simulink model "VCMGCM1962020b_v2"  (R2020b)
settings: Solver=FixedStepDiscrete  StartTime=0.0  StopTime=10.0  FixedStep=0.005  RelTol=1e-3  EnableMultiTasking=on
PreLoadFcn:
  | try, model_open; catch, disp('Error occurred while executing model pre-load callback: model_open.m'); disp('Please assure that the MATLAB working directory is set to the model directory before opening.'); end
InitFcn:
  | try, model_open; catch, end
undefined symbols (not defined in the file): Bridge, GCM, H, raptor_get_param_eval, raptor_get_safe_string, raptor_xcp_function
libraries: Blocks_lib x1165, Raptor_lib x665, simulink x62, VCM_lib x5
(part 14 of 23)

== system VCMGCM1962020b_v2/Fgnd/Virtual Sensors/Charger/Off Board/OffBoardChgr ==
  Data : Inport
  Bus Selector : BusSelector  OutputSignals=Sensors.CAN.CCS.CCSM2IEV_Command.CCSChargerType.CCSChargerType [Enum]
  Header : Blocks_lib/Header  width=Portrait  addtext=''
  SMART_DC : simulink/Logic and Bit Operations/Compare To Constant  relop===  const=3  OutDataTypeStr=boolean
  Bool : Outport  VectorParamsAs1DForOutWhenUnconnected=off
  wires:
  Data/1 -> Bus Selector/1
  Bus Selector/1 -> SMART_DC/1  "<CCSChargerType [Enum]>"
  SMART_DC/1 -> Bool/1

== system VCMGCM1962020b_v2/Fgnd/Virtual Sensors/Charger/Off Board/OffBoardChgrIsoFault ==
  Data : Inport
  Bus Selector : BusSelector  OutputSignals=Sensors.CAN.CCS.CCSEVSE_DC_ChargeInfo1.CCSEVSEIsolationStatus.CCSEVSEIsolationStatusVld [Bool],Sensors.CAN.CCS.CCSEVSE_DC_ChargeInfo1.CCSEVSEIsolationStatus.CCSEVSEIsolationStatus [Enum]
  Fault : simulink/Logic and Bit Operations/Compare To Constant  relop===  const=2  OutDataTypeStr=boolean
  Header : Blocks_lib/Header  width=Portrait  addtext=''
  Zero-Order Hold : ZeroOrderHold  SampleTime=-1
  Vld : Outport  VectorParamsAs1DForOutWhenUnconnected=off
  Bool : Outport  Port=2  VectorParamsAs1DForOutWhenUnconnected=off
  wires:
  Fault/1 -> Bool/1
  Bus Selector/2 -> Fault/1  "<CCSEVSEIsolationStatus [Enum]>"
  Data/1 -> Bus Selector/1
  Zero-Order Hold/1 -> Vld/1
  Bus Selector/1 -> Zero-Order Hold/1  "<CCSEVSEIsolationStatusVld [Bool]>"

== system VCMGCM1962020b_v2/Fgnd/Virtual Sensors/Charger/Off Board/OffBoardChgrShutdown ==
  Data : Inport
  Bus Selector : BusSelector  OutputSignals=Sensors.CAN.CCS.CCSEVSE_DC_ChargeInfo1.CCSEVSEStatusCode.CCSEVSEStatusCode [Enum]
  EVSE Shutdown : simulink/Logic and Bit Operations/Compare To Constant  relop===  const=2  OutDataTypeStr=boolean
  Header : Blocks_lib/Header  width=Portrait  addtext=''
  Bool : Outport  VectorParamsAs1DForOutWhenUnconnected=off
  wires:
  EVSE Shutdown/1 -> Bool/1
  Data/1 -> Bus Selector/1
  Bus Selector/1 -> EVSE Shutdown/1  "<CCSEVSEStatusCode [Enum]>"

== system VCMGCM1962020b_v2/Fgnd/Virtual Sensors/Charger/On Board/OnBoardChgr ==
  note: TBC
  Data : Inport
  BASIC_AC : simulink/Logic and Bit Operations/Compare To Constant  relop===  const=1  OutDataTypeStr=boolean
  Bus Selector : BusSelector  Commented=on  OutputSignals=Sensors.CAN.CCS.CCSM2IEV_Command.CCSChargerType.CCSChargerType [Enum]
  Constant : Constant
  Header : Blocks_lib/Header  width=Portrait  addtext=''
  Bool : Outport  VectorParamsAs1DForOutWhenUnconnected=off
  wires:
  Data/1 -> Bus Selector/1
  BASIC_AC/1 -> Bool/1
  Constant/1 -> BASIC_AC/1

== system VCMGCM1962020b_v2/Fgnd/Virtual Sensors/Charger/On Board/OnBoardChgrFault ==
  Data : Inport
  Bus Selector1 : BusSelector  OutputSignals=Sensors.CAN.OnBoardChgr.ChgrCCSA.ChgrCCSAMsgVld [Bool],Sensors.CAN.OnBoardChgr.ChgrCCSA.ChgrChrgr_hardware_protect.ChgrChrgr_hardware_protect [enum],Sensors.CAN.OnBoardChgr.ChgrCCSA.ChgrChargr_temp_flag.ChgrChargr_temp_flag [enum],Sensors.CAN.OnBoardChgr.ChgrCCSA.ChgrChrgr_input_volt_flag.ChgrChrgr_input_volt_flag [enum],Sensors.CAN.OnBoardChgr.ChgrCCSA.ChgrChrgr_input_volt_flag.ChgrChrgr_input_volt_flag [enum],Sensors.CAN.OnBoardChgr.ChgrCCSA.ChgrChrgr_input_volt_flag.ChgrChrgr_input_volt_flag [enum]
  CntrSat : Blocks_lib/CntrSat  init=0  inc=1  typ=uint16  relop=>=  th_nam='OnBoardChgrFaultVldWaitTime'  th_gain=samptime  th_units='sec'  th_help='On-board charger fault valid wait time'  th_group='Virtual Sensors | Charger'
  Header : Blocks_lib/Header  width=Portrait  addtext=''
  Logical Operator1 : Logic  OutDataTypeStr=boolean
  Logical Operator2 : Logic  Operator=NOT  Inputs=1  OutDataTypeStr=boolean
  Logical Operator3 : Logic  Operator=OR  Inputs=5  OutDataTypeStr=boolean
  Vld : Outport  VectorParamsAs1DForOutWhenUnconnected=off
  Bool : Outport  Port=2  VectorParamsAs1DForOutWhenUnconnected=off
  wires:
  Data/1 -> Bus Selector1/1
  Bus Selector1/1 -> Vld/1, Logical Operator1/1  "<ChgrCCSAMsgVld [Bool]>"
  Logical Operator2/1 -> CntrSat/2
  Logical Operator1/1 -> Logical Operator2/1, CntrSat/1
  CntrSat/1 -> Bool/1
  Logical Operator3/1 -> Logical Operator1/2
  Bus Selector1/2 -> Logical Operator3/1  "<ChgrChrgr_hardware_protect [enum]>"
  Bus Selector1/3 -> Logical Operator3/2  "<ChgrChargr_temp_flag [enum]>"
  Bus Selector1/4 -> Logical Operator3/3  "<ChgrChrgr_input_volt_flag [enum]>"
  Bus Selector1/5 -> Logical Operator3/4  "<ChgrChrgr_input_volt_flag [enum]>"
  Bus Selector1/6 -> Logical Operator3/5  "<ChgrChrgr_input_volt_flag [enum]>"

== system VCMGCM1962020b_v2/Fgnd/Virtual Sensors/Driver Inputs/APP/Learn-Up Enable ==
  Data : Inport
  Bus Selector : BusSelector  OutputSignals=VirtualSensors.Spd.VehSpd [kph]
  Header : Blocks_lib/Header  width=Portrait  addtext=''
  Relational Operator : RelationalOperator  Operator=<=  OutDataTypeStr=boolean  RndMeth=Nearest
  raptor_adjustment : Raptor_lib/Data Storage/raptor_adjustment  paramName='APPLearnUpEnblVehSpdThr'  nameSource=Parameter  initValue=0  dataType=double  storage=Calibration  calDispType=Number  calEnum={}  calGain=1.0  calOffset=0.0  calMax=inf  calMin=-inf  calFormat='-1'  calUnit='kph'  calHelp='Learn-up strategy enable vehicle speed threshold'  calAccess=1  calFunction='Virtual Sensors | Driver Input'  calDispHeaders=off  calColHeaders={'Col1' 'Col2' 'Col3'}  calRowHeaders={'Row1' 'Row2' 'Row3'}
      settings: SourceProductName=Raptor
  Bool : Outport  VectorParamsAs1DForOutWhenUnconnected=off
  wires:
  Bus Selector/1 -> Relational Operator/1  "<VehSpd [kph]>"
  Data/1 -> Bus Selector/1
  Relational Operator/1 -> Bool/1
  raptor_adjustment/1 -> Relational Operator/2

== system VCMGCM1962020b_v2/Fgnd/Virtual Sensors/Driver Inputs/Brk/BrkPos ==
  Data : Inport
  Arb : Blocks_lib/Arb  nam='BrkPos'  units='%'  eqn='(u(1) + u(2)) / 2'  minmax=min  samptime=samptime
  Bus Selector : BusSelector  OutputSignals=Sensors.Sensors.Driver.BrkPos1.BrkPos1Vld [Bool],Sensors.Sensors.Driver.BrkPos2.BrkPos2Vld [Bool],Sensors.Sensors.Driver.BrkPos1.BrkPos1 [%],Sensors.Sensors.Driver.BrkPos2.BrkPos2 [%]
  Bus Selector2 : BusSelector  OutputSignals=Sensors.Sensors.Driver.APP1.APP1Vld [Bool],Sensors.Sensors.Driver.APP1ADC [ADC]
  Bus Selector3 : BusSelector  OutputSignals=Sensors.Sensors.Driver.APP2.APP2Vld [Bool],Sensors.Sensors.Driver.APP2ADC [ADC]
  Ddbnd(PctInpt) : Blocks_lib/Ddbnd(PctInpt)  nam='BrkPos'  group='Virtual Sensors | Driver Input'
  Header : Blocks_lib/Header  width=Portrait  addtext=''
  Learn-Up Enable : Subsystem
  Meas&Ovrd : Blocks_lib/Meas&Ovrd  nam='BrkPos'  name_source=Parameter  view_as=Number  enum_struct={}  gain=1  min=-inf  max=inf  precision=''  units='%'  help='Accelerator pedal position'  group='Virtual Sensors | Driver Input'
  SnsLinPctAdapt : Blocks_lib/SnsLinPctAdapt  nam='BrkPos1'  group='Virtual Sensors | Driver Input'  samptime=samptime
  SnsLinPctAdapt1 : Blocks_lib/SnsLinPctAdapt  nam='BrkPos2'  group='Virtual Sensors | Driver Input'  samptime=samptime
  Vld : Outport  VectorParamsAs1DForOutWhenUnconnected=off
  % : Outport  Port=2  VectorParamsAs1DForOutWhenUnconnected=off
  wires:
  Data/1 -> Bus Selector3/1, Learn-Up Enable/1(Data), Bus Selector2/1, Bus Selector/1
  Arb/1 -> Vld/1
  Meas&Ovrd/1 -> %/1
  Bus Selector3/2 -> SnsLinPctAdapt1/2  "<APP2ADC [ADC]>"
  Bus Selector3/1 -> SnsLinPctAdapt1/1  "<APP2Vld [Bool]>"
  Learn-Up Enable/1(Bool) -> SnsLinPctAdapt1/3, SnsLinPctAdapt/3
  Bus Selector2/2 -> SnsLinPctAdapt/2  "<APP1ADC [ADC]>"
  Bus Selector2/1 -> SnsLinPctAdapt/1  "<APP1Vld [Bool]>"
  Bus Selector/4 -> Arb/4  "<BrkPos2 [%]>"
  Bus Selector/3 -> Arb/3  "<BrkPos1 [%]>"
  Bus Selector/2 -> Arb/2  "<BrkPos2Vld [Bool]>"
  Bus Selector/1 -> Arb/1  "<BrkPos1Vld [Bool]>"
  Arb/2 -> Ddbnd(PctInpt)/1
  Ddbnd(PctInpt)/1 -> Meas&Ovrd/1

== system VCMGCM1962020b_v2/Fgnd/Virtual Sensors/PDU/HVBusVolt/HV Bus Voltage ==
  Data : Inport
  Avg : Subsystem
  Demux : Demux
  Diag : Subsystem
  Function-Call Generator : simulink/Ports & Subsystems/Function-Call Generator  sample_time=-1  numberOfIterations=1  DisallowWideOutput=off
  Header : Blocks_lib/Header  width=Portrait  addtext=''
  Reset : Subsystem
  "Sum, Max, Min" : Subsystem
  Vld : Outport  VectorParamsAs1DForOutWhenUnconnected=off
  V : Outport  Port=2  VectorParamsAs1DForOutWhenUnconnected=off
  wires:
  Function-Call Generator/1 -> Demux/1
  Demux/2 -> "Sum, Max, Min"/Trigger
  Demux/3 -> Avg/Trigger
  Demux/4 -> Diag/Trigger
  Demux/1 -> Reset/Trigger
  Avg/2(V) -> Diag/1(V), V/1
  Avg/1(Vld) -> Vld/1
  Data/1 -> "Sum, Max, Min"/1(Data)

== system VCMGCM1962020b_v2/Fgnd/Virtual Sensors/Vehicle/Range/CntrLoop ==
  Compare To Constant : simulink/Logic and Bit Operations/Compare To Constant  relop=>=  const=rstval  OutDataTypeStr=boolean
  Constant : Constant  Value=init  OutDataTypeStr=uint16
  Header : Blocks_lib/Header  width=Portrait  addtext=''
  Increment Real World : simulink/Additional Math & Discrete/Additional Math: Increment - Decrement/Increment Real World
      settings: SourceProductBaseCode=SL
  Multiport Switch : MultiPortSwitch  DataPortOrder=Zero-based contiguous  Inputs=2  zeroidx=on  InputSameDT=on
  Unit Delay : UnitDelay  InitialCondition=init  SampleTime=-1  HasFrameUpgradeWarning=on
  Count : Outport  VectorParamsAs1DForOutWhenUnconnected=off
  wires:
  Constant/1 -> Multiport Switch/3
  Increment Real World/1 -> Multiport Switch/2
  Compare To Constant/1 -> Multiport Switch/1
  Multiport Switch/1 -> Unit Delay/1, Count/1
  Unit Delay/1 -> Compare To Constant/1, Increment Real World/1

== system VCMGCM1962020b_v2/Fgnd/Virtual Sensors/Vehicle/Range/RangeGain ==
  Odom : Inport
  data : Inport  Port=2
  Rst : Inport  Port=3
  Init : Inport  Port=4
  Enable : EnablePort
  Add : Sum  Inputs=+-
  Add2 : Sum  Inputs=-+
  Bus Selector : BusSelector  OutputSignals=VirtualSensors.Batt.BattSOC [%]
  Bus Selector1 : BusSelector  OutputSignals=Control.Mode.StartStop.RunMode [Bool]
  CntrLoop : Subsystem  TreatAsAtomicUnit=on  mask(CntrLoop){init=0, typ=uint16, rstval=2000}
      mask prompts: init "Initial Value"; typ "Data Type"; rstval "Reset at:"
      mask init:
      | cb = gcb;
      | 
      | % --- Parameter Setting
      | set_param([cb '/Constant'], 'OutDataTypeStr', typ);
      mask TypeOptions typ: double | single | int8 | uint8 | int16 | uint16 | int32 | uint32 | boolean
      mask Display: disp(['Loop Counter\nReset at ' num2str(rstval)]);
  Compare To Constant : simulink/Logic and Bit Operations/Compare To Constant  relop=~=  const=0  OutDataTypeStr=boolean
  Header : Blocks_lib/Header  width=Portrait  addtext=''
  Moving Average : Subsystem
  Mux : Mux  Inputs=2
  Saturation : Saturate  UpperLimit=100  LowerLimit=0
  Subsystem : Subsystem
  Unit Delay : UnitDelay  SampleTime=-1  HasFrameUpgradeWarning=on
  Unit Delay1 : UnitDelay  SampleTime=-1  HasFrameUpgradeWarning=on
  raptor_measurement : Raptor_lib/Data Storage/raptor_measurement  paramName='RangeEstTsTestpoint'  nameSource=Parameter  calDispType=Number  calEnum={'False', 'True'}  calGain=1.0  calOffset=0.0  calMax=inf  calMin=-inf  calFormat='-1'  calUnit='nd'  calHelp='Test point to determine how often the range estimate executes'  calAccess=1  calFunction='Virtual Sensors | Speed'  calVisible=on
      settings: SourceProductName=Raptor
  DOdomDSoc : Outport
  MvAv : Outport  Port=2
  wires:
  Odom/1 -> Unit Delay/1, Add/1
  Unit Delay1/1 -> Add2/2
  Bus Selector/1 -> Unit Delay1/1, Add2/1  "<BattSOC [%]>"
  Unit Delay/1 -> Add/2
  Add/1 -> Mux/1
  Add2/1 -> Saturation/1
  Moving Average/1(MvAv) -> MvAv/1
  Saturation/1 -> Compare To Constant/1, Mux/2
  Subsystem/1(Out1) -> Moving Average/1(In1), DOdomDSoc/1
  Mux/1 -> Subsystem/1(y)
  data/1 -> Bus Selector1/1, Bus Selector/1
  Compare To Constant/1 -> Subsystem/Enable
  Bus Selector1/1 -> Moving Average/2(In2)  "<RunMode [Bool]>"
  Rst/1 -> Moving Average/3(Rst)
  Init/1 -> Moving Average/4(Init)
  CntrLoop/1(Count) -> raptor_measurement/1

== system VCMGCM1962020b_v2/Fgnd/Virtual Sensors/Vehicle/Range/Subsystem1 ==
  Ground : Ground
  Header : Blocks_lib/Header  width=Portrait  addtext=''
  Meas&Ovrd1 : Blocks_lib/Meas&Ovrd  nam='RangeGainRst'  name_source=Parameter  view_as=Number  enum_struct={ 'no Reset' 'reset'}  gain=1  min=0  max=1  precision=''  units='Bool'  help='SOC Range Parameter reset'  group='Virtual Sensors | Speed'
  Multiport Switch : MultiPortSwitch  DataPortOrder=Zero-based contiguous  Inputs=2  DiagnosticForDefault=None  zeroidx=on
  Unit Delay : UnitDelay  SampleTime=-1  HasFrameUpgradeWarning=on
  raptor_adjustment : Raptor_lib/Data Storage/raptor_adjustment  paramName='RangeGainRst_Cal'  nameSource=Parameter  initValue=0.00  dataType=double  storage=Calibration  calDispType=Number  calEnum={'False', 'True'}  calGain=1.0  calOffset=0.0  calMax=inf  calMin=-inf  calFormat='-1'  calUnit='km/%SOC'  calHelp='Reset Value of the range gain parm'  calAccess=1  calFunction='Virtual Sensors | Speed'  calDispHeaders=off  calColHeaders={'Col1' 'Col2' 'Col3'}  calRowHeaders={'Row1' 'Row2' 'Row3'}
      settings: SourceProductName=Raptor
  raptor_data_def : Raptor_lib/Data Storage/raptor_data_def  dataName='RangeGainInit'  initValue=0  dataType=double  storage=NonVolatile (EEPROM)  calVisible=on  calType=Measurement  calDispType=Number  calEnum={'False', 'True'}  calGain=1.0  calOffset=0  calMin=-inf  calMax=inf  calFormat='-1'  calUnit='km/%SOC'  calHelp='The vehicle trip distance initial Odom at reset'  calAccess=1  calFunction='Virtual Sensors | Speed'  calDispHeaders=off  calColHeaders={'Col1' 'Col2' 'Col3'}  calRowHeaders={'Row1' 'Row2' 'Row3'}
      settings: SourceProductName=Raptor
  raptor_data_read : Raptor_lib/Data Storage/raptor_data_read  dataName='RangeGainInit'  dataShape=Scalar  idxSource=Input  idxRow=1  idxCol=1
      settings: SourceProductName=Raptor
  Rst : Outport
  Init : Outport  Port=2
  wires:
  Multiport Switch/1 -> Init/1
  Ground/1 -> Meas&Ovrd1/1
  Meas&Ovrd1/1 -> Multiport Switch/1, Rst/1
  raptor_data_read/1 -> Unit Delay/1
  raptor_adjustment/1 -> Multiport Switch/3
  Unit Delay/1 -> Multiport Switch/2

== system VCMGCM1962020b_v2/Fgnd/Virtual Sensors/Vehicle/VehOdmtr/Subsystem ==
  Odom : Inport
  <Trip_Reset [enum]> : Inport  Port=2
  Add : Sum  Inputs=+-
  Compare To Constant : simulink/Logic and Bit Operations/Compare To Constant  relop=<  const=0  OutDataTypeStr=boolean
  Header : Blocks_lib/Header  width=Portrait  addtext=''
  Multiport Switch : MultiPortSwitch  DataPortOrder=Zero-based contiguous  Inputs=2  DataPortForDefault=Additional data port  zeroidx=on
  OR : Logic  Operator=OR  AllPortsSameDT=off  OutDataTypeStr=boolean
  Saturation : Saturate  UpperLimit=100000  LowerLimit=0
  Unit Delay1 : UnitDelay  SampleTime=-1  HasFrameUpgradeWarning=on
  raptor_data_def : Raptor_lib/Data Storage/raptor_data_def  dataName='TripDistInit'  initValue=0  dataType=double  storage=NonVolatile (EEPROM)  calVisible=on  calType=Measurement  calDispType=Number  calEnum={'False', 'True'}  calGain=1.0  calOffset=0  calMin=-inf  calMax=inf  calFormat='-1'  calUnit='km'  calHelp='The vehicle trip distance initial Odom at reset'  calAccess=1  calFunction='Virtual Sensors | Speed'  calDispHeaders=off  calColHeaders={'Col1' 'Col2' 'Col3'}  calRowHeaders={'Row1' 'Row2' 'Row3'}
      settings: SourceProductName=Raptor
  raptor_data_read : Raptor_lib/Data Storage/raptor_data_read  dataName='TripDistInit'  dataShape=Scalar  idxSource=Input  idxRow=1  idxCol=1
      settings: SourceProductName=Raptor
  raptor_data_write : Raptor_lib/Data Storage/raptor_data_write  dataName='TripDistInit'  dataShape=Scalar  idxSource=Input Port  idxRow=1  idxCol=1
      settings: SourceProductName=Raptor
  raptor_measurement1 : Raptor_lib/Data Storage/raptor_measurement  paramName='TripDst'  nameSource=Parameter  calDispType=Number  calEnum={'Disabled', 'Enabled'}  calGain=1  calOffset=0  calMax=inf  calMin=-inf  calFormat=''  calUnit='km'  calHelp='Vehicle odometer trip distance'  calAccess=1  calFunction='Virtual Sensors | Speed'  calVisible=on
      settings: SourceProductName=Raptor
  Trip : Outport
  wires:
  Multiport Switch/1 -> Add/2, raptor_data_write/1
  <Trip_Reset [enum]>/1 -> OR/2
  Odom/1 -> Add/1, Multiport Switch/3
  Add/1 -> Unit Delay1/1, Saturation/1
  Saturation/1 -> raptor_measurement1/1, Trip/1  "TripDist [km]"
  Compare To Constant/1 -> OR/1
  OR/1 -> Multiport Switch/1
  raptor_data_read/1 -> Multiport Switch/4, Multiport Switch/2
  Unit Delay1/1 -> Compare To Constant/1

== system VCMGCM1962020b_v2/Fgnd/Virtual Sensors/Vehicle/VehSpd/Motor Speed-Based ==
  Data : Inport
  Bus Selector : BusSelector  OutputSignals=VirtualSensors.DrvInvtr.DrvMtrSpdVld [Bool]
  Bus Selector1 : BusSelector  OutputSignals=VirtualSensors.DrvInvtr.DrvMtrSpd [rpm]
  Eqn(w/DvdByZeroPro) : Blocks_lib/Eqn(w//DvdByZeroPro)  eqn='abs(u(1)) * u(2) * pi * 60 / (1000 * u(3))'  dmn='(1000 * u(3))'  dfltval=0
  Header : Blocks_lib/Header  width=Portrait  addtext=''
  Mux : Mux  Inputs=3
  raptor_adjustment : Raptor_lib/Data Storage/raptor_adjustment  paramName='WhlDia'  nameSource=Parameter  initValue=0  dataType=double  storage=Calibration  calDispType=Number  calEnum={'Disabled', 'Enabled'}  calGain=1  calOffset=0  calMax=inf  calMin=-inf  calFormat=''  calUnit='m'  calHelp='Wheel diameter'  calAccess=1  calFunction='Virtual Sensors | Speed'  calDispHeaders=off  calColHeaders={'Col1' 'Col2' 'Col3'}  calRowHeaders={'Row1' 'Row2' 'Row3'}
      settings: SourceProductName=Raptor
  raptor_adjustment1 : Raptor_lib/Data Storage/raptor_adjustment  paramName='MtrGearRatio'  nameSource=Parameter  initValue=0  dataType=double  storage=Calibration  calDispType=Number  calEnum={'Disabled', 'Enabled'}  calGain=1  calOffset=0  calMax=inf  calMin=-inf  calFormat=''  calUnit='-'  calHelp='Motor gear ratio (combined gear box and rear differential)'  calAccess=1  calFunction='Virtual Sensors | Speed'  calDispHeaders=off  calColHeaders={'Col1' 'Col2' 'Col3'}  calRowHeaders={'Row1' 'Row2' 'Row3'}
      settings: SourceProductName=Raptor
  raptor_measurement : Raptor_lib/Data Storage/raptor_measurement  paramName='VehSpdMtrSpdBased'  nameSource=Parameter  calDispType=Number  calEnum={'Disabled', 'Enabled'}  calGain=1  calOffset=0  calMax=inf  calMin=-inf  calFormat=''  calUnit='kph'  calHelp='Vehicle speed (motor speed-based)'  calAccess=1  calFunction='Virtual Sensors | Speed'  calVisible=on
      settings: SourceProductName=Raptor
  Vld : Outport  VectorParamsAs1DForOutWhenUnconnected=off
  Spd [kph] : Outport  Port=2  VectorParamsAs1DForOutWhenUnconnected=off
  tag scope: WheelDiam=global
  wires:
  Eqn(w/DvdByZeroPro)/1 -> Spd [kph]/1, raptor_measurement/1
  Mux/1 -> Eqn(w/DvdByZeroPro)/1
  Bus Selector1/1 -> Mux/1  "<DrvMtrSpd [rpm]>"
  raptor_adjustment1/1 -> Mux/3
  Data/1 -> Bus Selector/1, Bus Selector1/1
  Bus Selector/1 -> Vld/1  "<DrvMtrSpdVld [Bool]>"
  raptor_adjustment/1 -> [WheelDiam], Mux/2

== system VCMGCM1962020b_v2/Fgnd/Virtual Sensors/Vehicle/VehSpd/WSS Based ==
  In1 : Inport
  AND : Logic  AllPortsSameDT=off  OutDataTypeStr=boolean
  Bus Selector : BusSelector  OutputSignals=Sensors.Sensors.Other.WSS1.WSS1Vld [Bool],Sensors.Sensors.Other.WSS2.WSS2Vld [Bool],Sensors.Sensors.Other.WSS2.WSS2 [RPM],Sensors.Sensors.Other.WSS1.WSS1 [RPM]
  Constant : Constant  Value=pi*60/1000
  Divide : Product  Inputs=***
  Sum : Sum
  Vld : Outport
  Spd [kph] : Outport  Port=2
  wires:
  In1/1 -> Bus Selector/1
  Bus Selector/1 -> AND/1  "<WSS1Vld [Bool]>"
  AND/1 -> Vld/1
  Bus Selector/2 -> AND/2  "<WSS2Vld [Bool]>"
  Bus Selector/3 -> Sum/1  "<WSS2 [RPM]>"
  Bus Selector/4 -> Sum/2  "<WSS1 [RPM]>"
  Sum/1 -> Divide/1
  [WheelDiam] -> Divide/2
  Constant/1 -> Divide/3
  Divide/1 -> Spd [kph]/1

== system VCMGCM1962020b_v2/Fgnd/Actuators/CAN/Battery/ChgrBatt_State_Transition_Cmd/MsgTx ==
  note: TBC: Initiate ISO diagnostics during initial startup
  Data : Inport
  Enable : EnablePort
  Bus Selector : BusSelector  OutputSignals=Control.Mode.StartStop.MainCntrReq [Bool],Control.Mode.StartStop.RampDown [Bool]
  CANTxField : Blocks_lib/CANTxField  custom=on  custom_nam=[nam '---']  custom_units='---'
  CANTxField1 : Blocks_lib/CANTxField  custom=on  custom_nam=[nam '---']  custom_units='---'
  CANTxField2 : Blocks_lib/CANTxField  custom=on  custom_nam=[nam '---']  custom_units='---'
  Ground : Ground
  Header : Blocks_lib/Header  width=Landscape  addtext=''
  doublestrike : Subsystem
  raptor_can_txmsg : Raptor_lib/CAN/raptor_can_txmsg  canDefinition=struct('dbcFile', 'BMS dbc file_rev6.0.dbc','message', 'Batt_State_Transition_Cmd','comment', '','signals', {{'HiVolt_Bus_Connect_Cmd','Power_Down_Cmd','ISO_Test_Check'}},'enabled', [ 1 1 1;],'scaled', [ 1 1 1;],'canBus', 'bus','messageID', [ 203158363;],'idMask', [ 536870911;],'payloadMask', [],'payloadValue', [],'period', [ 20;],'mailbox', '''''','queueSize', [ 1;],'label', [ 1;],'ver', [ 2;],'showID', [ 0;],'showRaw', [ 0;],'fill', [ 0;],'editID', [ 0;],'signalOrder', [ 3;],'signalAscDes', [ 1;])  canBus=bus  queueSize=1  payloadMask=[]  payloadValue=[]  period=20  showID=0  label=1  idMask=hex2dec('1FFFFFFF')  fill=0  id=203158363  showRaw=0  signalOrder=3  signalInfo={{struct('Name', 'HiVolt_Bus_Connect_Cmd','Startbit', [ 0;],'SignalSize', [ 2;],'ByteOrder', 'LittleEndian','ValueType', 'UNSIGNED','Class', 'uint8','Signed', [ 0;],'Factor', [ 1;],'Offset', [ 0;],'Min', [ 0;],'Max', [ 3;],'Units', 'enum','Comment', '','StartBit', [ 0;]),struct('Name', 'Power_Down_Cmd','Startbit', [ 0;],'SignalSize', [ 2;],'ByteOrder', 'LittleEndian','ValueType', 'UNSIGNED','Class', 'uint8','Signed', [ 0;],'Factor', [ 1;],'Offset', [ 0;],'Min', [ 0;],'Max', [ 3;],'Units', 'enum','Comment', '','StartBit', [ 2;]),struct('Name', 'ISO_Test_Check','Startbit', [ 0;],'SignalSize', [ 2;],'ByteOrder', 'LittleEndian','ValueType', 'UNSIGNED','Class', 'uint8','Signed', [ 0;],'Factor', [ 1;],'Offset', [ 0;],'Min', [ 0;],'Max', [ 0;],'Units', 'enum','Comment', '','StartBit', [ 6;])}}
      settings: SourceProductName=Raptor
  wires:
  Bus Selector/1 -> CANTxField/1  "<MainCntrReq [Bool]>"
  Data/1 -> Bus Selector/1
  CANTxField2/1 -> raptor_can_txmsg/3  "ISO_Test_Check"
  CANTxField1/1 -> raptor_can_txmsg/2  "Power_Down_Cmd"
  Bus Selector/2 -> CANTxField1/1  "<RampDown [Bool]>"
  Ground/1 -> CANTxField2/1
  doublestrike/1(HiVolt_Bus_Connect_Cmd1) -> raptor_can_txmsg/1  "HiVolt_Bus_Connect_Cmd"
  CANTxField/1 -> doublestrike/1(<MainCntrReq [Bool]>)

== system VCMGCM1962020b_v2/Fgnd/Actuators/CAN/Battery/MsgName/MsgTx ==
  Data : Inport
  Enable : EnablePort
  Bus Selector : BusSelector  OutputSignals=Control.Chgr.OnBoardChgrEnblReq [Bool]
  CANTxField : Blocks_lib/CANTxField  custom=on  custom_nam=[nam '---']  custom_units='---'
  Header : Blocks_lib/Header  width=Landscape  addtext=''
  raptor_can_txmsg : Raptor_lib/CAN/raptor_can_txmsg  canDefinition=struct('dbcFile', 'BMS dbc file_rev6.0.dbc','message', 'BCH1','comment', '','signals', {{'Charger_Connect'}},'enabled', [ 1;],'scaled', [ 1;],'canBus', 'bus','messageID', [ 419239241;],'idMask', [ 536870911;],'payloadMask', [],'payloadValue', [],'period', [ 1000;],'mailbox', '''''','queueSize', [ 1;],'label', [ 1;],'ver', [ 2;],'showID', [ 0;],'showRaw', [ 0;],'fill', [ 0;],'editID', [ 0;],'signalOrder', [ 3;],'signalAscDes', [ 1;])  canBus=bus  queueSize=1  payloadMask=[]  payloadValue=[]  period=1000  showID=0  label=1  idMask=hex2dec('1FFFFFFF')  fill=0  id=419239241  showRaw=0  signalOrder=3  signalInfo={{struct('Name', 'Charger_Connect','Startbit', [ 0;],'SignalSize', [ 2;],'ByteOrder', 'LittleEndian','ValueType', 'UNSIGNED','Class', 'uint8','Signed', [ 0;],'Factor', [ 1;],'Offset', [ 0;],'Min', [ 0;],'Max', [ 3;],'Units', '','Comment', '','StartBit', [ 4;])}}
      settings: SourceProductName=Raptor
  wires:
  Bus Selector/1 -> CANTxField/1  "<OnBoardChgrEnblReq [Bool]>"
  CANTxField/1 -> raptor_can_txmsg/1  "Charger_Connect"
  Data/1 -> Bus Selector/1

== system VCMGCM1962020b_v2/Fgnd/Actuators/CAN/Body Control/BCMBCH1/MsgTx ==
  Data : Inport
  Enable : EnablePort
  Bus Selector : BusSelector  OutputSignals=VirtualSensors.Chgr.OnBoard.OnBoardChgrFault [Bool],Control.Mode.StartStop.ChgMode [Bool]
  Bus Selector1 : BusSelector  OutputSignals=VirtualSensors.Chgr.OnBoard.OnBoardChgrDCVolt [V]
  Bus Selector2 : BusSelector  OutputSignals=VirtualSensors.Chgr.OnBoard.OnBoardChgrOutCur [A]
  CANTxField : Blocks_lib/CANTxField  custom=on  custom_nam=[nam '---']  custom_units='---'
  CANTxField1 : Blocks_lib/CANTxField  custom=on  custom_nam=[nam '---']  custom_units='---'
  CANTxField2 : Blocks_lib/CANTxField  custom=on  custom_nam=[nam '---']  custom_units='---'
  Constant : Constant  Value=uint8(3)
  Header : Blocks_lib/Header  width=Landscape  addtext=''
  Switch : Switch  Criteria=u2 > Threshold
  raptor_can_txmsg : Raptor_lib/CAN/raptor_can_txmsg  canDefinition=struct('dbcFile', 'BCM_dbc_file_rev_9.1.dbc','message', 'BCH1','comment', '','signals', {{'Batt_Charger1_State','Batt_Charger_Output_Volt','Batt_Charger_Output_Curr'}},'enabled', [ 1 1 1;],'scaled', [ 1 1 1;],'canBus', 'bus','messageID', [ 419239407;],'idMask', [ 536870911;],'payloadMask', [],'payloadValue', [],'period', [ 100;],'mailbox', '''''','queueSize', [ 1;],'label', [ 1;],'ver', [ 2;],'showID', [ 0;],'showRaw', [ 0;],'fill', [ 0;],'editID', [ 0;],'signalOrder', [ 3;],'signalAscDes', [ 1;])  canBus=bus  queueSize=1  payloadMask=[]  payloadValue=[]  period=100  showID=0  label=1  idMask=hex2dec('1FFFFFFF')  fill=0  id=419239407  showRaw=0  signalOrder=3  signalInfo={{struct('Name', 'Batt_Charger1_State','Startbit', [ 0;],'SignalSize', [ 4;],'ByteOrder', 'LittleEndian','ValueType', 'UNSIGNED','Class', 'uint8','Signed', [ 0;],'Factor', [ 1;],'Offset', [ 0;],'Min', [ 0;],'Max', [ 15;],'Units', 'enum','Comment', '','StartBit', [ 0;]),struct('Name', 'Batt_Charger_Output_Volt','Startbit', [ 0;],'SignalSize', [ 16;],'ByteOrder', 'LittleEndian','ValueType', 'UNSIGNED','Class', 'uint16','Signed', [ 0;],'Factor', [ 0.05;],'Offset', [ 0;],'Min', [ 0;],'Max', [ 3212.75;],'Units', 'V','Comment', '','StartBit', [ 8;]),struct('Name', 'Batt_Charger_Output_Curr','Startbit', [ 0;],'SignalSize', [ 16;],'ByteOrder', 'LittleEndian','ValueType', 'UNSIGNED','Class', 'uint16','Signed', [ 0;],'Factor', [ 0.05;],'Offset', [ -1600;],'Min', [ -1600;],'Max', [ 1612.75;],'Units', 'A','Comment', '','StartBit', [ 24;])}}
      settings: SourceProductName=Raptor
  wires:
  CANTxField/1 -> raptor_can_txmsg/1  "Batt_Charger1_State"
  Data/1 -> Bus Selector2/1, Bus Selector1/1, Bus Selector/1
  Switch/1 -> CANTxField/1
  Bus Selector/1 -> Switch/2  "<OnBoardChgrFault [Bool]>"
  Bus Selector/2 -> Switch/3  "<ChgMode [Bool]>"
  Constant/1 -> Switch/1
  CANTxField1/1 -> raptor_can_txmsg/2  "Batt_Charger_Output_Volt"
  Bus Selector1/1 -> CANTxField1/1  "<OnBoardChgrDCVolt [V]>"
  CANTxField2/1 -> raptor_can_txmsg/3  "Batt_Charger_Output_Curr"
  Bus Selector2/1 -> CANTxField2/1  "<OnBoardChgrOutCur [A]>"

== system VCMGCM1962020b_v2/Fgnd/Actuators/CAN/Body Control/BCMCCVS1_VCU/MsgTx ==
  Data : Inport
  Enable : EnablePort
  Bus Selector : BusSelector  OutputSignals=VirtualSensors.Spd.VehSpd [kph]
  CANTxField : Blocks_lib/CANTxField  custom=on  custom_nam=[nam '---']  custom_units='---'
  Header : Blocks_lib/Header  width=Landscape  addtext=''
  raptor_can_txmsg : Raptor_lib/CAN/raptor_can_txmsg  canDefinition=struct('dbcFile', 'BCM_dbc_file_rev_9.1.dbc','message', 'CCVS1_VCU','comment', '','signals', {{'Whl_Veh_Spd','Brake_Switch'}},'enabled', [ 1 0;],'scaled', [ 1 1;],'canBus', 'bus','messageID', [ 419361263;],'idMask', [ 536870911;],'payloadMask', [],'payloadValue', [],'period', [ 100;],'mailbox', '''''','queueSize', [ 1;],'label', [ 1;],'ver', [ 2;],'showID', [ 0;],'showRaw', [ 0;],'fill', [ 0;],'editID', [ 0;],'signalOrder', [ 3;],'signalAscDes', [ 1;])  canBus=bus  queueSize=1  payloadMask=[]  payloadValue=[]  period=100  showID=0  label=1  idMask=hex2dec('1FFFFFFF')  fill=0  id=419361263  showRaw=0  signalOrder=3  signalInfo={{struct('Name', 'Whl_Veh_Spd','Startbit', [ 0;],'SignalSize', [ 16;],'ByteOrder', 'LittleEndian','ValueType', 'UNSIGNED','Class', 'uint16','Signed', [ 0;],'Factor', [ 0.0039063;],'Offset', [ 0;],'Min', [ 0;],'Max', [ 250.996;],'Units', 'kph','Comment', '','StartBit', [ 8;]),struct('Name', 'Brake_Switch','Startbit', [ 0;],'SignalSize', [ 2;],'ByteOrder', 'LittleEndian','ValueType', 'UNSIGNED','Class', 'uint8','Signed', [ 0;],'Factor', [ 1;],'Offset', [ 0;],'Min', [ 0;],'Max', [ 3;],'Units', 'enum','Comment', '','StartBit', [ 28;])}}
      settings: SourceProductName=Raptor
  wires:
  CANTxField/1 -> raptor_can_txmsg/1  "Whl_Veh_Spd"
  Data/1 -> Bus Selector/1
  Bus Selector/1 -> CANTxField/1  "<VehSpd [kph]>"

== system VCMGCM1962020b_v2/Fgnd/Actuators/CAN/Body Control/BCMCM3/MsgTx ==
  Enable : EnablePort
  CANTxField : Blocks_lib/CANTxField  custom=on  custom_nam=[nam '---']  custom_units='---'
  Constant : Constant  Value=uint8(3)
  Header : Blocks_lib/Header  width=Landscape  addtext=''
  raptor_can_txmsg : Raptor_lib/CAN/raptor_can_txmsg  canDefinition=struct('dbcFile', 'BCM_dbc_file_rev_9.1.dbc','message', 'CM3','comment', '','signals', {{'Veh_Trailer_Status'}},'enabled', [ 1;],'scaled', [ 1;],'canBus', 'bus','messageID', [ 419288303;],'idMask', [ 536870911;],'payloadMask', [],'payloadValue', [],'period', [ 100;],'mailbox', '''''','queueSize', [ 1;],'label', [ 1;],'ver', [ 2;],'showID', [ 0;],'showRaw', [ 0;],'fill', [ 0;],'editID', [ 0;],'signalOrder', [ 3;],'signalAscDes', [ 1;])  canBus=bus  queueSize=1  payloadMask=[]  payloadValue=[]  period=100  showID=0  label=1  idMask=hex2dec('1FFFFFFF')  fill=0  id=419288303  showRaw=0  signalOrder=3  signalInfo={{struct('Name', 'Veh_Trailer_Status','Startbit', [ 0;],'SignalSize', [ 2;],'ByteOrder', 'LittleEndian','ValueType', 'UNSIGNED','Class', 'uint8','Signed', [ 0;],'Factor', [ 1;],'Offset', [ 0;],'Min', [ 0;],'Max', [ 3;],'Units', 'enum','Comment', '','StartBit', [ 12;])}}
      settings: SourceProductName=Raptor
  wires:
  CANTxField/1 -> raptor_can_txmsg/1  "Veh_Trailer_Status"
  Constant/1 -> CANTxField/1

== system VCMGCM1962020b_v2/Fgnd/Actuators/CAN/Body Control/BCMETC2/MsgTx ==
  Data : Inport
  Enable : EnablePort
  Bus Selector : BusSelector  OutputSignals=Control.Mode.PRNDMode_Act [enum]
  CANTxField : Blocks_lib/CANTxField  custom=on  custom_nam=[nam '---']  custom_units='---'
  Header : Blocks_lib/Header  width=Landscape  addtext=''
  raptor_can_txmsg : Raptor_lib/CAN/raptor_can_txmsg  canDefinition=struct('dbcFile', 'BCM_dbc_file_rev_9.1.dbc','message', 'ETC2','comment', '','signals', {{'Trans_curr_gear'}},'enabled', [ 1;],'scaled', [ 1;],'canBus', 'bus','messageID', [ 418383343;],'idMask', [ 536870911;],'payloadMask', [],'payloadValue', [],'period', [ 100;],'mailbox', '''''','queueSize', [ 1;],'label', [ 1;],'ver', [ 2;],'showID', [ 0;],'showRaw', [ 0;],'fill', [ 0;],'editID', [ 0;],'signalOrder', [ 3;],'signalAscDes', [ 1;])  canBus=bus  queueSize=1  payloadMask=[]  payloadValue=[]  period=100  showID=0  label=1  idMask=hex2dec('1FFFFFFF')  fill=0  id=418383343  showRaw=0  signalOrder=3  signalInfo={{struct('Name', 'Trans_curr_gear','Startbit', [ 0;],'SignalSize', [ 8;],'ByteOrder', 'LittleEndian','ValueType', 'SIGNED','Class', 'int8','Signed', [ 1;],'Factor', [ 1;],'Offset', [ 0;],'Min', [ -125;],'Max', [ 125;],'Units', '1 gear value / bit','Comment', '','StartBit', [ 32;])}}
      settings: SourceProductName=Raptor
  wires:
  CANTxField/1 -> raptor_can_txmsg/1  "Trans_curr_gear"
  Data/1 -> Bus Selector/1
  Bus Selector/1 -> CANTxField/1  "<PRNDMode_Act [enum]>"

== system VCMGCM1962020b_v2/Fgnd/Actuators/CAN/Body Control/BCMICMSTS/MsgTx ==
  Data : Inport
  Enable : EnablePort
  Bus Selector : BusSelector  OutputSignals=Sensors.Sensors.Volt.Wake [Bool]
  CANTxField : Blocks_lib/CANTxField  custom=off  custom_nam=[nam '---']  custom_units='---'
  Constant : Constant  Value=uint8(0)
  Constant1 : Constant  Value=uint8(4)
  Header : Blocks_lib/Header  width=Landscape  addtext=''
  Switch : Switch  Criteria=u2 > Threshold
  raptor_can_txmsg : Raptor_lib/CAN/raptor_can_txmsg  canDefinition=struct('dbcFile', 'BCM_dbc_file_rev_9.1.dbc','message', 'ICMSTS','comment', '','signals', {{'VCU_Ign_Stat'}},'enabled', [ 1;],'scaled', [ 1;],'canBus', 'bus','messageID', [ 419213807;],'idMask', [ 536870911;],'payloadMask', [],'payloadValue', [],'period', [ 100;],'mailbox', '''''','queueSize', [ 1;],'label', [ 1;],'ver', [ 2;],'showID', [ 0;],'showRaw', [ 0;],'fill', [ 0;],'editID', [ 0;],'signalOrder', [ 3;],'signalAscDes', [ 1;])  canBus=bus  queueSize=1  payloadMask=[]  payloadValue=[]  period=100  showID=0  label=1  idMask=hex2dec('1FFFFFFF')  fill=0  id=419213807  showRaw=0  signalOrder=3  signalInfo={{struct('Name', 'VCU_Ign_Stat','Startbit', [ 0;],'SignalSize', [ 3;],'ByteOrder', 'LittleEndian','ValueType', 'UNSIGNED','Class', 'uint8','Signed', [ 0;],'Factor', [ 1;],'Offset', [ 0;],'Min', [ 0;],'Max', [ 7;],'Units', 'enum','Comment', '','StartBit', [ 0;])}}
      settings: SourceProductName=Raptor
  wires:
  CANTxField/1 -> raptor_can_txmsg/1  "VCU_Ign_Stat"
  Data/1 -> Bus Selector/1
  Bus Selector/1 -> Switch/2  "<Wake [Bool]>"
  Constant/1 -> Switch/3
  Constant1/1 -> Switch/1
  Switch/1 -> CANTxField/1

== system VCMGCM1962020b_v2/Fgnd/Actuators/CAN/Body Control/BCMVEP2/MsgTx ==
  Data : Inport
  Enable : EnablePort
  Bus Selector : BusSelector  OutputSignals=Sensors.Sensors.Volt.DRVPVolt.DRVPVolt [V]
  CANTxField : Blocks_lib/CANTxField  custom=on  custom_nam=[nam '---']  custom_units='---'
  Header : Blocks_lib/Header  width=Landscape  addtext=''
  raptor_can_txmsg : Raptor_lib/CAN/raptor_can_txmsg  canDefinition=struct('dbcFile', 'BCM_dbc_file_rev_9.1.dbc','message', 'VEP2','comment', '','signals', {{'Low_Voltage_System_Voltage'}},'enabled', [ 1;],'scaled', [ 1;],'canBus', 'bus','messageID', [ 419335663;],'idMask', [ 536870911;],'payloadMask', [],'payloadValue', [],'period', [ 100;],'mailbox', '''''','queueSize', [ 1;],'label', [ 1;],'ver', [ 2;],'showID', [ 0;],'showRaw', [ 0;],'fill', [ 0;],'editID', [ 0;],'signalOrder', [ 3;],'signalAscDes', [ 1;])  canBus=bus  queueSize=1  payloadMask=[]  payloadValue=[]  period=100  showID=0  label=1  idMask=hex2dec('1FFFFFFF')  fill=0  id=419335663  showRaw=0  signalOrder=3  signalInfo={{struct('Name', 'Low_Voltage_System_Voltage','Startbit', [ 0;],'SignalSize', [ 16;],'ByteOrder', 'LittleEndian','ValueType', 'UNSIGNED','Class', 'uint16','Signed', [ 0;],'Factor', [ 0.05;],'Offset', [ 0;],'Min', [ 0;],'Max', [ 3212.75;],'Units', 'V','Comment', '','StartBit', [ 0;])}}
      settings: SourceProductName=Raptor
  wires:
  CANTxField/1 -> raptor_can_txmsg/1  "Low_Voltage_System_Voltage"
  Data/1 -> Bus Selector/1
  Bus Selector/1 -> CANTxField/1  "<DRVPVolt [V]>"

== system VCMGCM1962020b_v2/Fgnd/Actuators/CAN/Body Control/MsgName/MsgTx ==
  Data : Inport
  Enable : EnablePort
  Bus Selector : BusSelector  OutputSignals=Control.Mode.StartStop.RunMode [Bool]
  CANTxField : Blocks_lib/CANTxField  custom=on  custom_nam=[nam '---']  custom_units='---'
  Constant : Constant
  Constant1 : Constant  Value=4
  Header : Blocks_lib/Header  width=Landscape  addtext=''
  Multiport Switch : MultiPortSwitch  DataPortOrder=Zero-based contiguous  Inputs=2  zeroidx=on
  raptor_can_txmsg : Raptor_lib/CAN/raptor_can_txmsg  canDefinition=struct('dbcFile', 'BCM_dbc_file_rev_9.0.dbc','message', 'ICMSTS','comment', '','signals', {{'VCU_Ign_Stat'}},'enabled', [ 1;],'scaled', [ 1;],'canBus', 'bus','messageID', [ 419213807;],'idMask', [ 536870911;],'payloadMask', [],'payloadValue', [],'period', [ 100;],'mailbox', '''''','queueSize', [ 1;],'label', [ 1;],'ver', [ 2;],'showID', [ 0;],'showRaw', [ 0;],'fill', [ 0;],'editID', [ 0;],'signalOrder', [ 3;],'signalAscDes', [ 1;])  canBus=bus  queueSize=1  payloadMask=[]  payloadValue=[]  period=100  showID=0  label=1  idMask=hex2dec('1FFFFFFF')  fill=0  id=419213807  showRaw=0  signalOrder=3  signalInfo={{struct('Name', 'VCU_Ign_Stat','Startbit', [ 0;],'SignalSize', [ 3;],'ByteOrder', 'LittleEndian','ValueType', 'UNSIGNED','Class', 'uint8','Signed', [ 0;],'Factor', [ 1;],'Offset', [ 0;],'Min', [ 0;],'Max', [ 7;],'Units', 'enum','Comment', '','StartBit', [ 0;])}}
      settings: SourceProductName=Raptor
  wires:
  CANTxField/1 -> raptor_can_txmsg/1  "VCU_Ign_Stat"
  Data/1 -> Bus Selector/1
  Bus Selector/1 -> Multiport Switch/1  "<RunMode [Bool]>"
  Multiport Switch/1 -> CANTxField/1
  Constant/1 -> Multiport Switch/2
  Constant1/1 -> Multiport Switch/3

== system VCMGCM1962020b_v2/Fgnd/Actuators/CAN/CCS Interface/CCSEV_ChargeParameters1/MsgTx ==
  Data : Inport
  Enable : EnablePort
  EVEnergyRequest : Subsystem
      settings: OpenFcn=open_system(gcb,'force')
  Header : Blocks_lib/Header  width=Landscape  addtext=''
  raptor_adjustment : Raptor_lib/Data Storage/raptor_adjustment  paramName=[nam 'EVMaximumCurrentLimit']  nameSource=Parameter  initValue=400  dataType=double  storage=Calibration  calDispType=Number  calEnum={'False', 'True'}  calGain=1.0  calOffset=0.0  calMax=inf  calMin=-inf  calFormat='-1'  calUnit='A'  calHelp='EV maximum current limit'  calAccess=1  calFunction=['Actuators | CAN | ' msgnam]  calDispHeaders=off  calColHeaders={'Col1' 'Col2' 'Col3'}  calRowHeaders={'Row1' 'Row2' 'Row3'}
      settings: SourceProductName=Raptor
  raptor_adjustment1 : Raptor_lib/Data Storage/raptor_adjustment  paramName=[nam 'EVMaximumPowerLimit']  nameSource=Parameter  initValue=300  dataType=double  storage=Calibration  calDispType=Number  calEnum={'False', 'True'}  calGain=1.0  calOffset=0.0  calMax=inf  calMin=-inf  calFormat='-1'  calUnit='kW'  calHelp='EV maximum power limit'  calAccess=1  calFunction=['Actuators | CAN | ' msgnam]  calDispHeaders=off  calColHeaders={'Col1' 'Col2' 'Col3'}  calRowHeaders={'Row1' 'Row2' 'Row3'}
      settings: SourceProductName=Raptor
  raptor_adjustment2 : Raptor_lib/Data Storage/raptor_adjustment  paramName=[nam 'EVMaximumVoltageLimit']  nameSource=Parameter  initValue=765  dataType=double  storage=Calibration  calDispType=Number  calEnum={'False', 'True'}  calGain=1.0  calOffset=0.0  calMax=inf  calMin=-inf  calFormat='-1'  calUnit='V'  calHelp='EV maximum voltage limit'  calAccess=1  calFunction=['Actuators | CAN | ' msgnam]  calDispHeaders=off  calColHeaders={'Col1' 'Col2' 'Col3'}  calRowHeaders={'Row1' 'Row2' 'Row3'}
      settings: SourceProductName=Raptor
  raptor_can_txmsg : Raptor_lib/CAN/raptor_can_txmsg  canDefinition=struct('dbcFile', 'm2iev-api.dbc','message', 'EV_ChargeParameters1','comment', 'EV_ChargeParameters1','signals', {{'EVMaximumCurrentLimit','EVMaximumPowerLimit','EVMaximumVoltageLimit','EVEnergyRequest'}},'enabled', [ 1 1 1 1;],'canBus', 'bus','messageID', [ 512;],'idMask', [ 536870911;],'payloadMask', [],'payloadValue', [],'period', [ 1000;],'mailbox', '''''','queueSize', [ 1;],'label', [ 1;],'ver', [ 2;],'showID', [ 0;],'showRaw', [ 0;],'fill', [ 0;],'editID', [ 0;],'signalOrder', [ 3;])  canBus=bus  queueSize=1  payloadMask=[]  payloadValue=[]  period=1000  showID=0  label=1  idMask=hex2dec('1FFFFFFF')  fill=0  id=512  showRaw=0  signalOrder=3  signalInfo={{struct('Name', 'EVMaximumCurrentLimit','Startbit', [ 0;],'SignalSize', [ 16;],'ByteOrder', 'LittleEndian','ValueType', 'SIGNED','Class', 'int16','Signed', [ 1;],'Factor', [ 0.05;],'Offset', [ 0;],'Min', [ -1638.4;],'Max', [ 1638.35;],'Units', 'A','Comment', 'Maximim current EV may request from EVSE','StartBit', [ 0;]),struct('Name', 'EVMaximumPowerLimit','Startbit', [ 0;],'SignalSize', [ 16;],'ByteOrder', 'LittleEndian','ValueType', 'UNSIGNED','Class', 'uint16','Signed', [ 0;],'Factor', [ 0.05;],'Offset', [ 0;],'Min', [ 0;],'Max', [ 3276.75;],'Units', 'kW','Comment', 'Maximum power EV may request from EVSE','StartBit', [ 16;]),struct('Name', 'EVMaximumVoltageLimit','Startbit', [ 0;],'SignalSize', [ 16;],'ByteOrder', 'LittleEndian','ValueType', 'UNSIGNED','Class', 'uint16','Signed', [ 0;],'Factor', [ 0.05;],'Offset', [ 0;],'Min', [ 0;],'Max', [ 3276.75;],'Units', 'V','Comment', 'Maximum voltage EV may request from EVSE','StartBit', [ 32;]),struct('Name', 'EVEnergyRequest','Startbit', [ 0;],'SignalSize', [ 16;],'ByteOrder', 'LittleEndian','ValueType', 'UNSIGNED','Class', 'uint16','Signed', [ 0;],'Factor', [ 0.05;],'Offset', [ 0;],'Min', [ 0;],'Max', [ 3276.75;],'Units', 'kWh','Comment', 'Energy that EV wants to transfer into the battery','StartBit', [ 48;])}}
      settings: SourceProductName=Raptor
  wires:
  EVEnergyRequest/1(kWh) -> raptor_can_txmsg/4  "EVEnergyRequest"
  raptor_adjustment2/1 -> raptor_can_txmsg/3  "EVMaximumVoltageLimit"
  raptor_adjustment1/1 -> raptor_can_txmsg/2  "EVMaximumPowerLimit"
  raptor_adjustment/1 -> raptor_can_txmsg/1  "EVMaximumCurrentLimit"
  Data/1 -> EVEnergyRequest/1(Data)

== system VCMGCM1962020b_v2/Fgnd/Actuators/CAN/CCS Interface/CCSEV_ChargeParameters2/MsgTx ==
  Data : Inport
  Enable : EnablePort
  Header : Blocks_lib/Header  width=Landscape  addtext=''
  Terminator : Terminator
  raptor_adjustment : Raptor_lib/Data Storage/raptor_adjustment  paramName=[nam 'EnergyCapacity']  nameSource=Parameter  initValue=33  dataType=double  storage=Calibration  calDispType=Number  calEnum={'False', 'True'}  calGain=1.0  calOffset=0.0  calMax=inf  calMin=-inf  calFormat='-1'  calUnit='kWh'  calHelp='EV energy capacity'  calAccess=1  calFunction=['Actuators | CAN | ' msgnam]  calDispHeaders=off  calColHeaders={'Col1' 'Col2' 'Col3'}  calRowHeaders={'Row1' 'Row2' 'Row3'}
      settings: SourceProductName=Raptor
  raptor_adjustment1 : Raptor_lib/Data Storage/raptor_adjustment  paramName=[nam 'FullSOC']  nameSource=Parameter  initValue=0  dataType=double  storage=Calibration  calDispType=Number  calEnum={'False', 'True'}  calGain=1.0  calOffset=0.0  calMax=inf  calMin=-inf  calFormat='-1'  calUnit='%'  calHelp='Full SOC'  calAccess=1  calFunction=['Actuators | CAN | ' msgnam]  calDispHeaders=off  calColHeaders={'Col1' 'Col2' 'Col3'}  calRowHeaders={'Row1' 'Row2' 'Row3'}
      settings: SourceProductName=Raptor
  raptor_adjustment2 : Raptor_lib/Data Storage/raptor_adjustment  paramName=[nam 'BulkSOC']  nameSource=Parameter  initValue=0  dataType=double  storage=Calibration  calDispType=Number  calEnum={'False', 'True'}  calGain=1.0  calOffset=0.0  calMax=inf  calMin=-inf  calFormat='-1'  calUnit='%'  calHelp='Bulk SOC'  calAccess=1  calFunction=['Actuators | CAN | ' msgnam]  calDispHeaders=off  calColHeaders={'Col1' 'Col2' 'Col3'}  calRowHeaders={'Row1' 'Row2' 'Row3'}
      settings: SourceProductName=Raptor
  raptor_adjustment3 : Raptor_lib/Data Storage/raptor_adjustment  paramName=[nam 'AllowedACCharging']  nameSource=Parameter  initValue=0  dataType=boolean  storage=Calibration  calDispType=Number  calEnum={'False', 'True'}  calGain=1.0  calOffset=0.0  calMax=inf  calMin=-inf  calFormat='-1'  calUnit='Boolean'  calHelp='Allowed AC charging'  calAccess=1  calFunction=['Actuators | CAN | ' msgnam]  calDispHeaders=off  calColHeaders={'Col1' 'Col2' 'Col3'}  calRowHeaders={'Row1' 'Row2' 'Row3'}
      settings: SourceProductName=Raptor
  raptor_adjustment4 : Raptor_lib/Data Storage/raptor_adjustment  paramName=[nam 'AllowedSmartDCCharging']  nameSource=Parameter  initValue=0  dataType=boolean  storage=Calibration  calDispType=Number  calEnum={'False', 'True'}  calGain=1.0  calOffset=0.0  calMax=inf  calMin=-inf  calFormat='-1'  calUnit='Boolean'  calHelp='Allowed smart DC charging'  calAccess=1  calFunction=['Actuators | CAN | ' msgnam]  calDispHeaders=off  calColHeaders={'Col1' 'Col2' 'Col3'}  calRowHeaders={'Row1' 'Row2' 'Row3'}
      settings: SourceProductName=Raptor
  raptor_can_txmsg : Raptor_lib/CAN/raptor_can_txmsg  canDefinition=struct('dbcFile', 'm2iev-api.dbc','message', 'EV_ChargeParameters2','comment', 'EV_ChargeParameters2','signals', {{'EVEnergyCapacity','FullSOC','BulkSOC','AllowedACCharging','AllowedSmartDCCharging'}},'enabled', [ 1 1 1 1 1;],'canBus', 'bus','messageID', [ 513;],'idMask', [ 536870911;],'payloadMask', [],'payloadValue', [],'period', [ 1000;],'mailbox', '''''','queueSize', [ 1;],'label', [ 1;],'ver', [ 2;],'showID', [ 0;],'showRaw', [ 0;],'fill', [ 0;],'editID', [ 0;],'signalOrder', [ 3;])  canBus=bus  queueSize=1  payloadMask=[]  payloadValue=[]  period=1000  showID=0  label=1  idMask=hex2dec('1FFFFFFF')  fill=0  id=513  showRaw=0  signalOrder=3  signalInfo={{struct('Name', 'EVEnergyCapacity','Startbit', [ 0;],'SignalSize', [ 16;],'ByteOrder', 'LittleEndian','ValueType', 'UNSIGNED','Class', 'uint16','Signed', [ 0;],'Factor', [ 0.05;],'Offset', [ 0;],'Min', [ 0;],'Max', [ 3276.75;],'Units', 'kWh','Comment', 'Capacity of the EV`s battery pack','StartBit', [ 0;]),struct('Name', 'FullSOC','Startbit', [ 0;],'SignalSize', [ 8;],'ByteOrder', 'LittleEndian','ValueType', 'UNSIGNED','Class', 'uint8','Signed', [ 0;],'Factor', [ 0.5;],'Offset', [ 0;],'Min', [ 0;],'Max', [ 100;],'Units', '%','Comment', 'State of fully charged battery pack (must be 100%)','StartBit', [ 16;]),struct('Name', 'BulkSOC','Startbit', [ 0;],'SignalSize', [ 8;],'ByteOrder', 'LittleEndian','ValueType', 'UNSIGNED','Class', 'uint8','Signed', [ 0;],'Factor', [ 0.5;],'Offset', [ 0;],'Min', [ 0;],'Max', [ 100;],'Units', '%','Comment', 'Bulk charging threshold (e.g. 80%)','StartBit', [ 24;]),struct('Name', 'AllowedACCharging','Startbit', [ 0;],'SignalSize', [ 1;],'ByteOrder', 'LittleEndian','ValueType', 'UNSIGNED','Class', 'uint8','Signed', [ 0;],'Factor', [ 1;],'Offset', [ 0;],'Min', [ 0;],'Max', [ 1;],'Units', 'Boolean','Comment', 'Indication whether basic AC charging is allowed','StartBit', [ 43;]),struct('Name', 'AllowedSmartDCCharging','Startbit', [ 0;],'SignalSize', [ 1;],'ByteOrder', 'LittleEndian','ValueType', 'UNSIGNED','Class', 'uint8','Signed', [ 0;],'Factor', [ 1;],'Offset', [ 0;],'Min', [ 0;],'Max', [ 1;],'Units', 'Boolean','Comment', 'Indication whether smart DC charging is allowed','StartBit', [ 45;])}}
      settings: SourceProductName=Raptor
  wires:
  Data/1 -> Terminator/1
  raptor_adjustment4/1 -> raptor_can_txmsg/5  "AllowedSmartDCCharging"
  raptor_adjustment3/1 -> raptor_can_txmsg/4  "AllowedACCharging"
  raptor_adjustment/1 -> raptor_can_txmsg/1  "EVEnergyCapacity"
  raptor_adjustment1/1 -> raptor_can_txmsg/2  "FullSOC"
  raptor_adjustment2/1 -> raptor_can_txmsg/3  "BulkSOC"
